simulink library "sm_car_testrig_utilities_lib"  (R2022b)
settings: Solver=VariableStepAuto  StartTime=0.0  StopTime=10.0  RelTol=1e-3
undefined symbols (not defined in the file): Maneuver, tire_radius, Vehicle, Visual, X, Y, Z
libraries: sm_lib x31, nesl_utility x17, fl_lib x3, $bdroot x3, Tire_Utilities x2, Surface_Profile_Axle2_KnC x2, simulink x2
(part 2 of 2)

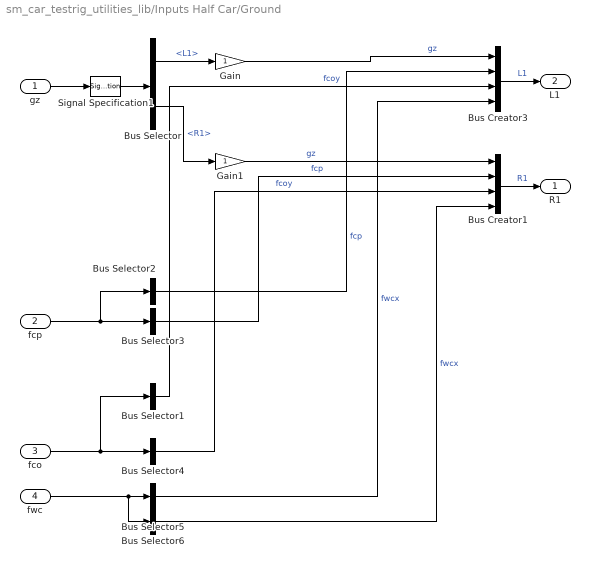
== system sm_car_testrig_utilities_lib/Inputs Half Car/Ground ==
  gz : Inport
  fcp : Inport  Port=2
  fco : Inport  Port=3
  fwc : Inport  Port=4
  Bus Creator1 : BusCreator  Inputs=4
  Bus Creator3 : BusCreator  Inputs=4
  Bus Selector : BusSelector  OutputSignals=L1,R1
  Bus Selector1 : BusSelector  OutputSignals=L1.fcoy  OutputAsBus=on
  Bus Selector2 : BusSelector  OutputSignals=L1.fx,L1.fy,L1.tz  OutputAsBus=on
  Bus Selector3 : BusSelector  OutputSignals=R1.fx,R1.fy,R1.tz  OutputAsBus=on
  Bus Selector4 : BusSelector  OutputSignals=R1.fcoy  OutputAsBus=on
  Bus Selector5 : BusSelector  OutputSignals=L1.fwcx  OutputAsBus=on
  Bus Selector6 : BusSelector  OutputSignals=R1.fwcx  OutputAsBus=on
  Gain : Gain
  Gain1 : Gain
  Signal Specification1 : SignalSpecification  Unit=m
  R1 : Outport  VectorParamsAs1DForOutWhenUnconnected=off
  L1 : Outport  Port=2  VectorParamsAs1DForOutWhenUnconnected=off
  wires:
  Bus Creator1/1 -> R1/1  "R1"
  Bus Creator3/1 -> L1/1  "L1"
  Signal Specification1/1 -> Bus Selector/1
  Bus Selector/1 -> Gain/1  "<L1>"
  gz/1 -> Signal Specification1/1
  Bus Selector/2 -> Gain1/1  "<R1>"
  Gain1/1 -> Bus Creator1/1  "gz"
  Gain/1 -> Bus Creator3/1  "gz"
  Bus Selector3/1 -> Bus Creator1/2  "fcp"
  fcp/1 -> Bus Selector2/1, Bus Selector3/1
  Bus Selector2/1 -> Bus Creator3/2  "fcp"
  fco/1 -> Bus Selector4/1, Bus Selector1/1
  Bus Selector1/1 -> Bus Creator3/3  "fcoy"
  Bus Selector4/1 -> Bus Creator1/3  "fcoy"
  fwc/1 -> Bus Selector6/1, Bus Selector5/1
  Bus Selector5/1 -> Bus Creator3/4  "fwcx"
  Bus Selector6/1 -> Bus Creator1/4  "fwcx"

== system sm_car_testrig_utilities_lib/Inputs Half Car/Logging RdBus ==
  L1 : Inport
  Bus Creator : BusCreator  Inputs=1
  Bus Creator1 : BusCreator  Inputs=3
  Bus Creator2 : BusCreator  Inputs=1
  Bus Selector : BusSelector  OutputSignals=L1.fx,L1.fy,L1.tz
  RdBus : Outport
  wires:
  Bus Selector/3 -> Bus Creator1/3  "<tz>"
  Bus Selector/2 -> Bus Creator1/2  "<fy>"
  Bus Selector/1 -> Bus Creator1/1  "<fx>"
  Bus Creator2/1 -> Bus Creator/1  "L1"
  Bus Creator1/1 -> Bus Creator2/1  "fcp"
  Bus Creator/1 -> RdBus/1
  L1/1 -> Bus Selector/1

== system sm_car_testrig_utilities_lib/Inputs Half Car/Steering ==
  Off : Subsystem  VariantControl=Off
  On : Subsystem  VariantControl=On
  qStr : Outport
  xRk : Outport  Port=2

== system sm_car_testrig_utilities_lib/Inputs Quarter Car/Logging RdBus ==
  L1 : Inport
  Bus Creator : BusCreator  Inputs=1
  Bus Creator1 : BusCreator  Inputs=3
  Bus Creator2 : BusCreator  Inputs=1
  Bus Selector : BusSelector  OutputSignals=L1.fx,L1.fy,L1.tz
  RdBus : Outport
  wires:
  L1/1 -> Bus Selector/1
  Bus Creator/1 -> RdBus/1
  Bus Creator1/1 -> Bus Creator2/1  "fcp"
  Bus Creator2/1 -> Bus Creator/1  "L1"
  Bus Selector/1 -> Bus Creator1/1  "<fx>"
  Bus Selector/2 -> Bus Creator1/2  "<fy>"
  Bus Selector/3 -> Bus Creator1/3  "<tz>"

== system sm_car_testrig_utilities_lib/Inputs Quarter Car/Steering ==
  Off : Subsystem  VariantControl=Off
  On : Subsystem  VariantControl=On
  qStr : Outport
  xRk : Outport  Port=2

== system sm_car_testrig_utilities_lib/Inputs Half Car/Steering/Off ==
  Constant : Constant  Value=0
  qStr : Outport
  xRk : Outport  Port=2
  wires:
  Constant/1 -> qStr/1, xRk/1

== system sm_car_testrig_utilities_lib/Inputs Half Car/Steering/On ==
  Steer to Rack : Lookup_n-D  NumberOfTableDimensions=1  BreakpointsForDimension1=Vehicle.Chassis.SuspA1.Steer.Ratio_Table.aWheel.Value  Table=Vehicle.Chassis.SuspA1.Steer.Ratio_Table.xRack.Value  InternalRulePriority=Speed  RndMeth=Simplest
  qSteer : simulink/Sources/Repeating Sequence  rep_seq_t=Maneuver.Steer.t.Value  rep_seq_y=Maneuver.Steer.aWheel.Value
  qStr : Outport
  xRk : Outport  Port=2
  wires:
  Steer to Rack/1 -> xRk/1
  qSteer/1 -> Steer to Rack/1, qStr/1

== system sm_car_testrig_utilities_lib/Inputs Quarter Car/Steering/Off ==
  Constant : Constant  Value=0
  qStr : Outport
  xRk : Outport  Port=2
  wires:
  Constant/1 -> xRk/1, qStr/1

== system sm_car_testrig_utilities_lib/Inputs Quarter Car/Steering/On ==
  Steer to Rack : Lookup_n-D  NumberOfTableDimensions=1  BreakpointsForDimension1=Vehicle.Chassis.SuspA1.Steer.Ratio_Table.aWheel.Value  Table=Vehicle.Chassis.SuspA1.Steer.Ratio_Table.xRack.Value  InternalRulePriority=Speed  RndMeth=Simplest
  qSteer : simulink/Sources/Repeating Sequence  rep_seq_t=Maneuver.Steer.t.Value  rep_seq_y=Maneuver.Steer.aWheel.Value
  qStr : Outport
  xRk : Outport  Port=2
  wires:
  qSteer/1 -> qStr/1, Steer to Rack/1
  Steer to Rack/1 -> xRk/1
